simulink model "ACtoAC"  (R2026a)
settings: Solver=ode23t  StopTime=0.05  MaxStep=0.001  RelTol=1e-6  AbsTol=1e-6  EnableMultiTasking=on
libraries: nesl_utility x35, fl_lib x34, ee_lib x17
CloseFcn:
  | try,close(h1_FullWaveBridgeRectifier),end
  | clear h1_FullWaveBridgeRectifier
  | 
  | 
  | clear simlog_FullWaveBridgeRectifier
Description:
  | Full-Wave Bridge Rectifier
settings Model: Creator=The MathWorks, Inc.  LastModifiedBy=MME
settings DebuggingCC: PregeneratedLibrarySubsystemCodeDiagnostic=none
settings HardwareCC: ProdHWDeviceType=32-bit Generic
settings SimscapeCC: SimscapeNominalValues="[{\"value\":\"1\",\"unit\":\"A\"},{\"value\":\"1\",\"unit\":\"bar\"},{\"value\":\"1\",\"unit\":\"cm^2\"},{\"value\":\"1\",\"unit\":\"cm^3/s\"},{\"value\":\"1\",\"unit\":\"kJ/kg\"},{\"value\":\"1\",\"unit\":\"kW\"},{\"value\":\"1\",\"unit\":\"l\"},{\"value\":\"1\",\"unit\":\"N\"},{\"value\":\"1\",\"unit\":\"N*m\"},{\"value\":\"1\",\"unit\":\"V\"}]"  SimscapeLogSimulationStatistics=on  SimscapeLogName=simlog_FullWaveBridgeRectifier

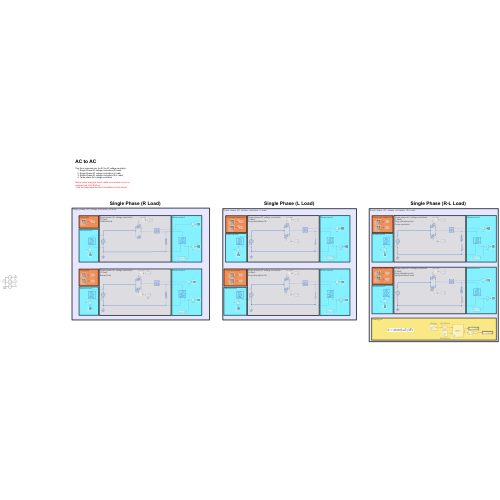
[thumbnail: Simulink's stored preview of the top-level diagram]
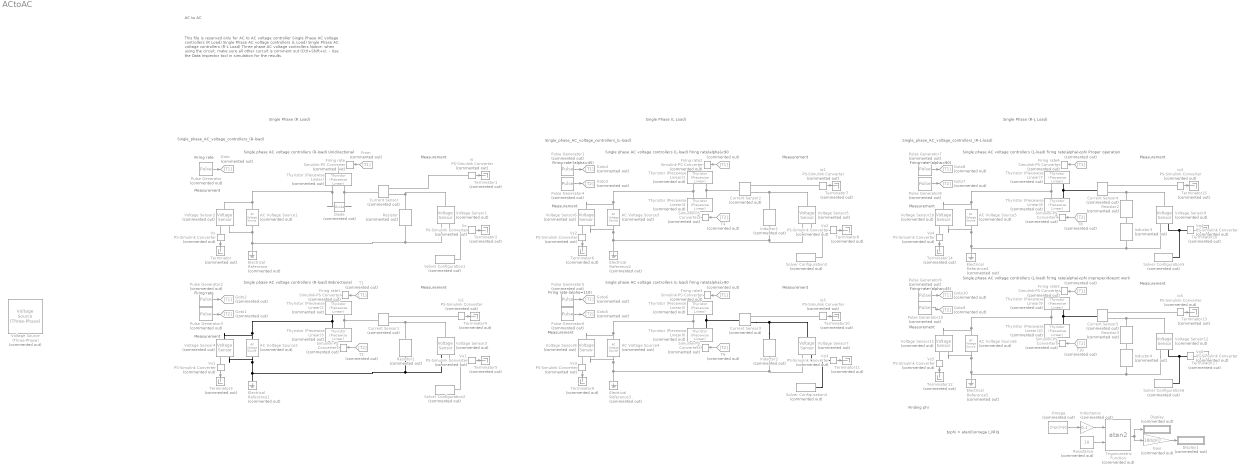
== system ACtoAC ==
  note: $\phi = atan((\omega L)/R)$
  note: Finding phi
  note: Single_phase_AC_voltage_controllers_(L-load)
  note: Single_phase_AC_voltage_controllers_(R-load)
  note: Measurement
  note: Firing rate
  note: Single phase AC voltage controllers
      | (R-load)
      | Unidirectional
  note: This file is reserved only for AC to AC voltage controller
      | Single Phase AC voltage controllers (R Load)
      | Single Phase AC voltage controllers (L Load)
      | Single Phase AC voltage controllers (R-L Load)
      | Three phase AC voltage controllers
      |
      | Notice: when using the circuit, make sure all other curcuit is comment out (Ctrl+Shift+x).
      | - Use the Data Inspector tool in simulation for the results.
  note: AC to AC
  note: Measurement
  note: Measurement
  note: Single phase AC voltage controllers
      | (R-load)
      | Bidirectional
  note: Firing rate
  note: Measurement
  note: Measurement
  note: Single phase AC voltage controllers
      | (L-load)
      | firing rate(alpha)<90
  note: Firing rate (alpha=45)
  note: Measurement
  note: Firing rate (alpha=110)
  note: Measurement
  note: Measurement
  note: Single phase AC voltage controllers
      | (L-load)
      | firing rate(alpha)>90
  note: Single Phase (R Load)
  note: Single Phase (L Load)
  note: Single Phase (R-L Load)
  note: Single_phase_AC_voltage_controllers_(R-L-load)
  note: Firing rate (alpha=90)
  note: Measurement
  note: Measurement
  note: Single phase AC voltage controllers
      | (L-load)
      | firing rate(alpha)<phi
      | Proper operation
  note: Single phase AC voltage controllers
      | (L-load)
      | firing rate(alpha)<phi
      | improper/doesnt work
  note: Measurement
  note: Firing rate (alpha=45)
  note: Measurement
  AC Voltage Source{1..6} (6 alike) : fl_lib/Electrical/Electrical Sources/AC Voltage Source  Commented=on  amp=120*sqrt(2) V  shift=0 deg  frequency=50 Hz
  Current Sensor{,1..5} (6 alike) : fl_lib/Electrical/Electrical Sensors/Current Sensor  Commented=on
  Diode : ee_lib/Semiconductors & Converters/Diode  Commented=on  ModelType=ee.enum.diode.modelType.pwl  TableType=ee.enum.diode.tableType.IfMat  IfMat=[.07, .12, .19, 1.75, 4.24, 7.32, 11.2; .16, .3, .72, 2.14, 5.02, 8.35, 13.12] A  VfMat=[.9, 1.15, 1.25, 1.5, 1.75, 2.17, 2.6, 2.85; .58, .68, .75, 1.1, 1.38, 1.77, 2.27, 2.7] V  TjVec=[25, 125] degC  VfVec=[.5, .7, .9, 1.3, 1.7, 2.1, 2.5] V  IfVec=[.1, .2, .5, 1, 2, 4, 7, 10] A  IrMat=[1e-06, 2e-06, 5e-06, 1e-05, 2.5e-05, 5e-05, .0001; 2e-06, 5e-06, 1e-05, 4e-05, 8e-05, .0002, .0005] A  VrMat=[10, 100, 200, 250, 300, 325, 350; 10, 70, 160, 220, 270, 300, 320] V  VrVec=[10, 20, 40, 50, 70, 80, 100] V  IrVec=[1e-06, 2e-06, 5e-06, 1e-05, 2e-05, 5e-05, .0001] A  Vf=0.6 V  Ron=0.3 Ohm  Goff=1e-8 S  prmExp=ee.enum.diode.expParam.useTwo  I12=[.0137, .545] A  V12=[.6, .7] V  RS=0 Ohm  Tmeas=298.15 K  IS=1e-12 A  ec=1  I1=0.0137 A  V1=0.6 V  N_series=1  N_parallel=1  ZenerEnable=false  Rz=0.3 Ohm  BV=30 V  C_param=ee.enum.diode.capParam.fixed  CJ=0 pF  CJ0=5 pF  Vvec=[.1, 10, 100] V  Cvec=[3.5, 1, .4] pF  VJ=1 V  Mgrad=0.5  FC=0.5  Q_param=ee.enum.diode.recoveryParam.off  iRM=-7.15 A  iF=4 A  didt=-750 A/us  trr_factor=3  trr=115 ns  Qrr=150 nA*s  Vr=-600 V  Ls=150 nH  Erec=0.03 J  TT=50 ns  tau=100 ns  T_param=ee.enum.diode.temperatureParam.off  Tdevice=298.15 K  I1_T2=0.245 A  V1_T2=0.5 V  IS_T2=1.25e-7 A  Tmeas2=125 degC  XTI_param=ee.enum.diode.xtiParam.pn  XTI=3  EG_param=ee.enum.diode.egapParam.material_si  EG=1.11 eV  dBVdT=0 V/K  enable_fault_input=simscape.enum.onoff.off  i_specify=off  i_priority=None  i=0 A  i_nominal_specify=off  i_nominal_value=1  i_nominal_unit=A  v_specify=off  v_priority=None  v=0 V  v_nominal_specify=off  v_nominal_value=1  v_nominal_unit=V  v_capacitor_specify=off  v_capacitor_priority=None  v_capacitor=0 V  v_capacitor_nominal_specify=off  v_capacitor_nominal_value=1  v_capacitor_nominal_unit=V  Qj_specify=off  Qj_priority=High  Qj=0 C  Qj_nominal_specify=off  Qj_nominal_value=1  Qj_nominal_unit=C  i_diode_specify=off  i_diode_priority=None  i_diode=0 A  i_diode_nominal_specify=off  i_diode_nominal_value=1  i_diode_nominal_unit=A  v_diode_specify=off  v_diode_priority=None  v_diode=0 V  v_diode_nominal_specify=off  v_diode_nominal_value=1  v_diode_nominal_unit=V  i_capacitor_specify=off  i_capacitor_priority=None  i_capacitor=0 A  i_capacitor_nominal_specify=off  i_capacitor_nominal_value=1  i_capacitor_nominal_unit=A  fidelity_level=ee.enum.diode.fidelity.includeChargeDyn  rec_loss_model=ee.enum.diode.reverseRecoveryModelTabulateUpTo3D.fixed  ErecVal=0 J  scaleWithIandV=true  ErecMat=zeros(2, 3) J  ErecMat3D=zeros(2, 3, 2) J  TjrecVec=[298.15, 398.15] K  IfrecVec=[.1, 1, 10] A  IrecVal=10 A  VrecVal=10 V  VrecVec=[0, 100] V  tFilter=1 / 1000 / 100 s  thermal_network_parameterization=ee.enum.thermalNetworkTopology.junctionCase  Rth=[0, 10] K/W  Rth_Cauer=[1, 3, 10] K/W  Rth_Foster=[.08, .14, .22, .16] K/W  thermal_mass_parameterization=ee.enum.thermalNetwork.timeconstant  thermal_mass=[0, 1] J/K  thermal_mass_Cauer=[.1, .3, 1] J/K  thermal_mass_Foster=[.001, .005, .05, .5] J/K  thermal_time_constant=[0, 10] s  thermal_time_constant_Cauer=[1, 3, 10] s  thermal_time_constant_Foster=[7e-05, .0007, .01, .08] s  thermal_mass_initial_temperatures=[25, 25] degC  thermal_mass_initial_temperatures_Cauer=[25, 25, 25] degC  junction_thermal_mass=0.01 J/K  Tvec_initial_Foster=[25, 25, 25, 25] degC  no_thermal_network=0  junction_temperature_specify=off  junction_temperature_priority=None  junction_temperature=25 degC  junction_temperature_nominal_specify=off  junction_temperature_nominal_value=1  junction_temperature_nominal_unit=degC
  Display : Display  Commented=on
  Display1 : Display  Commented=on
  Electrical Reference{,1..5} (6 alike) : fl_lib/Electrical/Electrical Elements/Electrical Reference  Commented=on
  Firing rate{,1..5} (6 alike) : nesl_utility/Simulink-PS Converter  Commented=on  PhysicalDomain=network_engine_domain  SubClassName=ps_input  LeftPortType=input  RightPortType=output  PseudoPeriodic=off  Frequencies=[]  NoiseDistribution=none  NoiseParameters=[]  Unit=1  AffineConversion=off  FilteringAndDerivatives=provide  SimscapeFilterOrder=1  InputFilterTimeConstant=0.001  UdotUserProvided=0
  From : From  Commented=on  GotoTag=T1
  Gain : Gain  Commented=on  Gain=180/pi()
  Goto{,2,4,6,8,10} (6 alike) : Goto  Commented=on  GotoTag=T1
  Goto{1,3,5,7,9} (5 alike) : Goto  Commented=on  GotoTag=T2
  Inductance : Gain  Commented=on  Gain=0.1
  Inductor{1..4} (4 alike) : ee_lib/Passive/Inductor  Commented=on  l=1e-1 H  enable_L_tol=ee.enum.toleranceApplication.none  L_tol=20  tol_distribution=ee.enum.toleranceDistribution.uniform  nSigma=4  r=0 Ohm  g=1e-9 1/Ohm  enable_operating_limits=ee.enum.enable.no  operating_limit_action=ee.enum.passive.reportOpLim.warn  max_working_current=1 A  power_rating=1 W  i_L_specify=off  i_L_priority=High  i_L=0 A  i_L_nominal_specify=off  i_L_nominal_value=1  i_L_nominal_unit=A
  Omega : Constant  Commented=on  Value=2*pi()*50
  Pulse Generator : DiscretePulseGenerator  Commented=on  PulseType=Time based  Amplitude=10  Period=0.02  PulseWidth=30  PhaseDelay=0.02*45/360
  Pulse Generator1 : DiscretePulseGenerator  Commented=on  PulseType=Time based  Amplitude=10  Period=0.02  PulseWidth=10  PhaseDelay=0.02*45/360
  Pulse Generator10 : DiscretePulseGenerator  Commented=on  PulseType=Time based  Amplitude=10  Period=0.02  PulseWidth=10  PhaseDelay=0.02*(70+180)/360
  Pulse Generator2 : DiscretePulseGenerator  Commented=on  PulseType=Time based  Amplitude=10  Period=0.02  PulseWidth=30  PhaseDelay=0.02*45/360
  Pulse Generator3 : DiscretePulseGenerator  Commented=on  PulseType=Time based  Amplitude=10  Period=0.02  PulseWidth=30  PhaseDelay=0.02*(45+180)/360
  Pulse Generator4 : DiscretePulseGenerator  Commented=on  PulseType=Time based  Amplitude=10  Period=0.02  PulseWidth=10  PhaseDelay=0.02*(45+180)/360
  Pulse Generator5 : DiscretePulseGenerator  Commented=on  PulseType=Time based  Amplitude=10  Period=0.02  PulseWidth=10  PhaseDelay=0.02*110/360
  Pulse Generator6 : DiscretePulseGenerator  Commented=on  PulseType=Time based  Amplitude=10  Period=0.02  PulseWidth=10  PhaseDelay=0.02*(110+180)/360
  Pulse Generator7 : DiscretePulseGenerator  Commented=on  PulseType=Time based  Amplitude=10  Period=0.02  PulseWidth=10  PhaseDelay=0.02*90/360
  Pulse Generator8 : DiscretePulseGenerator  Commented=on  PulseType=Time based  Amplitude=10  Period=0.02  PulseWidth=10  PhaseDelay=0.02*(90+180)/360
  Pulse Generator9 : DiscretePulseGenerator  Commented=on  PulseType=Time based  Amplitude=10  Period=0.02  PulseWidth=10  PhaseDelay=0.02*70/360
  Resistance : Constant  Commented=on  Value=10
  Resistor : fl_lib/Electrical/Electrical Elements/Resistor  Commented=on  R=1 Ohm  i_specify=off  i_priority=None  i=0 A  i_nominal_specify=off  i_nominal_value=1  i_nominal_unit=A  v_specify=off  v_priority=None  v=0 V  v_nominal_specify=off  v_nominal_value=1  v_nominal_unit=V
  Resistor1 : fl_lib/Electrical/Electrical Elements/Resistor  Commented=on  R=1 Ohm  i_specify=off  i_priority=None  i=0 A  i_nominal_specify=off  i_nominal_value=1  i_nominal_unit=A  v_specify=off  v_priority=None  v=0 V  v_nominal_specify=off  v_nominal_value=1  v_nominal_unit=V
  Resistor2 : fl_lib/Electrical/Electrical Elements/Resistor  Commented=on  R=10 Ohm  i_specify=off  i_priority=None  i=0 A  i_nominal_specify=off  i_nominal_value=1  i_nominal_unit=A  v_specify=off  v_priority=None  v=0 V  v_nominal_specify=off  v_nominal_value=1  v_nominal_unit=V
  Resistor3 : fl_lib/Electrical/Electrical Elements/Resistor  Commented=on  R=10 Ohm  i_specify=off  i_priority=None  i=0 A  i_nominal_specify=off  i_nominal_value=1  i_nominal_unit=A  v_specify=off  v_priority=None  v=0 V  v_nominal_specify=off  v_nominal_value=1  v_nominal_unit=V
  Simulink-PS Converter{1..5} (5 alike) : nesl_utility/Simulink-PS Converter  Commented=on  PhysicalDomain=network_engine_domain  SubClassName=ps_input  LeftPortType=input  RightPortType=output  PseudoPeriodic=off  Frequencies=[]  NoiseDistribution=none  NoiseParameters=[]  Unit=1  AffineConversion=off  FilteringAndDerivatives=provide  SimscapeFilterOrder=1  InputFilterTimeConstant=0.001  UdotUserProvided=0
  Solver Configuration{1..6} (6 alike) : nesl_utility/Solver Configuration  Commented=on  PhysicalDomain=network_engine_domain  SubClassName=solver  LeftPortType=input  RightPortType=generic  Tones=[]  Harmonics=[]  SimulateNoise=off  Profile=off  UseLocalSampling=off  EnableSwitchedLinearOptims=on  FrequencyDomain=off  UseCCode=off  RelTol=0.001  AbsTol=1e-06  MinStep=1e-09  ToWorkspace=off  RevertToSquareIcSolve=off  NumHomotopyIterations=100  PhasorMode=off  PhasorModeNumHarmonics=1  ConsistencySolver=NEWTON_XTOL_AFTER_FTOL  CanonicalOrdering=UNORDERED  OptimizeIntermediates=UNOPTIMIZED  IndexReductionMethod=DerivativeReplacement  DoDC=off  ResidualTolerance=1e-9  ConsistencyTolSource=GLOBAL  ConsistencyAbsTol=0.001  ConsistencyRelTol=0.001  ConsistencyTolFactor=0.001  UseLocalSolver=off  LocalSolverChoice=NE_BACKWARD_EULER_ADVANCER  ResolveIndetEquations=on  FunctionEvalNumThread=1  LocalSolverSampleTime=.001  DoFixedCost=off  MaxNonlinIter=3  MaxModeIter=2  ComputeImpulses=off  ImpulseIterations=2  LinearAlgebra=auto  LinearAlgebraNumThread=0  EquationFormulation=NE_TIME_EF  DelaysMemoryBudget=1024  AutomaticFiltering=on  FilteringTimeConstant=0.001  PartitionStorageMethod=AS_NEEDED  PartitionMemoryBudget=1024  PartitionMethod=FAST  MultibodyUseLocalSolver=off  MultibodyLocalSolverChoice=ODE1  MultibodyLocalSolverSampleTime=0.001
  T{1,3,5,7,9} (5 alike) : From  Commented=on  GotoTag=T1
  T{2,4,6,8,10} (5 alike) : From  Commented=on  GotoTag=T2
  Terminator{,1..17} (18 alike) : Terminator  Commented=on
  Thyristor (Piecewise Linear){,1..10} (11 alike) : ee_lib/Semiconductors & Converters/Thyristor (Piecewise Linear)  Commented=on  port_option=ee.enum.controlport.ps  Vf=0.8 V  Ron=0.001 Ohm  Goff=1e-5 1/Ohm  Vgt=6 V  Ih=1 A  diode_param=ee.enum.semiconductors.protectionDiode.external  diode_Vf=0.8 V  diode_Ron=0.001 Ohm  diode_Goff=1e-5 1/Ohm  diode_C=50e-9 F  diode_iRM=-235 A  diode_iF=300 A  diode_idot=-50 A/us  diode_trr_param=ee.enum.converters.diodetrr.trr_factor  diode_trr_factor=3  diode_trr=15 us  diode_Qrr=1500 s*uA  iak_specify=off  iak_priority=None  iak=0 A  iak_nominal_specify=off  iak_nominal_value=1  iak_nominal_unit=A  vak_specify=off  vak_priority=None  vak=0 V  vak_nominal_specify=off  vak_nominal_value=1  vak_nominal_unit=V  vgk_specify=off  vgk_priority=None  vgk=0 V  vgk_nominal_specify=off  vgk_nominal_value=1  vgk_nominal_unit=V  thermal_loss_option=ee.enum.converters.thermalLossOption.constantvalues  Von_data=[0, .1, .6, .8, 1, 1.3, 1.6, 2, 2.4; 0, .1, .7, 1, 1.2, 1.5, 1.9, 2.4, 2.8] V  Tj=[298.15, 398.15] K  Iout_data=[0, .1, 1, 5, 10, 20, 40, 70, 100] A  Eon_data=[0, .0024, .024, .12, .2, .48, 1.04, 2.16, 3.24; 0, .003, .03, .15, .25, .6, 1.3, 2.7, 4.05] * 1e-3 J  Tj_loss=[298.15, 398.15] K  Iout_data_loss=[0, .1, 1, 5, 10, 20, 40, 70, 100] A  Eon_scalar=22.86e-3 J  Eoff_natural_commutation=10e-3 J  Voff=300 V  Iout_scalar=600 A  onCurrentMeasDelay=1e-4 s  diodeModelType=ee.enum.converters.diodeModelType.pwl  diodeTableType=ee.enum.diode.tableType.IfMat  diode_IfMat=[.07, .12, .19, 1.75, 4.24, 7.32, 11.2; .16, .3, .72, 2.14, 4.02, 6.35, 9.12] A  diode_VfMat=[.9, 1.15, 1.25, 1.5, 1.75, 2.17, 2.6, 2.85; .58, .68, .75, 1.1, 1.38, 1.77, 2.27, 2.7] V  diode_TjVec=[25, 125] degC  diode_VfVec=[.5, .7, .9, 1.3, 1.7, 2.1, 2.5] V  diode_IfVec=[.1, .2, .5, 1, 2, 4, 7, 10] A  diode_rec_loss_model=ee.enum.diode.reverseRecoveryModel.fixed  diode_ErecVal=0 J  diode_scaleWithIandV=true  diode_ErecMat=zeros(2, 3) J  diode_TjrecVec=[298.15, 398.15] K  diode_IfrecVec=[.1, 1, 10] A  diode_IrecVal=10 A  diode_VrecVal=10 V  diode_tFilter=1 / 1000 / 100 s  thermal_network_parameterization=ee.enum.thermalNetworkTopology.external  Rth=[.08, .5] K/W  Rth_Cauer=[.08, .1, .5] K/W  Rth_Foster=[.08, .14, .22, .16] K/W  thermal_mass_parameterization=ee.enum.thermalNetwork.timeconstant  thermal_mass=[.01, .5] J/K  thermal_mass_Cauer=[.01, .1, .5] J/K  thermal_mass_Foster=[.001, .005, .05, .5] J/K  thermal_time_constant=[.001, .2] s  thermal_time_constant_Cauer=[.001, .1, .2] s  thermal_time_constant_Foster=[7e-05, .0007, .01, .08] s  thermal_mass_initial_temperatures=[25, 25] degC  thermal_mass_initial_temperatures_Cauer=[25, 25, 25] degC  junction_thermal_mass=0.01 J/K  Tvec_initial_Foster=[25, 25, 25, 25] degC  junction_temperature_specify=off  junction_temperature_priority=None  junction_temperature=25 degC  junction_temperature_nominal_specify=off  junction_temperature_nominal_value=1  junction_temperature_nominal_unit=degC  Qj_specify=off  Qj_priority=None  Qj=0 W  Qj_nominal_specify=off  Qj_nominal_value=1  Qj_nominal_unit=W  accumulatedSwitchingLosses_specify=off  accumulatedSwitchingLosses_priority=None  accumulatedSwitchingLosses=0 J
  Trigonometric Function : Trigonometry  Commented=on  Operator=atan2
  Vo{,1..5} (6 alike) : nesl_utility/PS-Simulink Converter  Commented=on  PhysicalDomain=network_engine_domain  SubClassName=ps_output  LeftPortType=input  RightPortType=output  PseudoPeriodic=off  Frequencies=[]  VectorFormat=inherit  Unit=inherit  AffineConversion=off
  Voltage Source (Three-Phase) : ee_lib/Sources/Voltage Source (Three-Phase)  Commented=on  vline_rms=sqrt(3) * 325 / sqrt(2) V  shift=0 deg  freq=50 Hz  impedance_option=1  SShortCircuit=1e6 A*V  XR=15  R=0.01 Ohm  L=3.97e-4 H  harmonic_option=0  harmonic_orders=[5, 7, 11, 13]  harmonic_ratios=[.1, .1, .1, .1]  G_parasitic=0 1/Ohm  I_specify=off  I_priority=None  I=[0, 0, 0] A  I_nominal_specify=off  I_nominal_value=1  I_nominal_unit=A
  Voltage Sensor{1..12} (12 alike) : fl_lib/Electrical/Electrical Sensors/Voltage Sensor  Commented=on
  Vs{,1..5} (6 alike) : nesl_utility/PS-Simulink Converter  Commented=on  PhysicalDomain=network_engine_domain  SubClassName=ps_output  LeftPortType=input  RightPortType=output  PseudoPeriodic=off  Frequencies=[]  VectorFormat=inherit  Unit=inherit  AffineConversion=off
  io{,1..5} (6 alike) : nesl_utility/PS-Simulink Converter  Commented=on  PhysicalDomain=network_engine_domain  SubClassName=ps_output  LeftPortType=input  RightPortType=output  PseudoPeriodic=off  Frequencies=[]  VectorFormat=inherit  Unit=inherit  AffineConversion=off
  wires:
  From/1 -> Firing rate/1
  Pulse Generator/1 -> Goto/1
  Vo/1 -> Terminator2/1
  io/1 -> Terminator1/1
  Vs/1 -> Terminator/1
  io1/1 -> Terminator4/1
  Vs1/1 -> Terminator3/1
  Pulse Generator3/1 -> Goto1/1
  T1/1 -> Firing rate1/1
  Vo1/1 -> Terminator5/1
  T2/1 -> Simulink-PS Converter1/1
  Pulse Generator2/1 -> Goto2/1
  Vo2/1 -> Terminator8/1
  T3/1 -> Firing rate2/1
  T4/1 -> Simulink-PS Converter2/1
  io2/1 -> Terminator7/1
  Vs2/1 -> Terminator6/1
  Pulse Generator4/1 -> Goto3/1
  Pulse Generator1/1 -> Goto4/1
  Vo3/1 -> Terminator11/1
  Pulse Generator6/1 -> Goto5/1
  Vs3/1 -> Terminator9/1
  T6/1 -> Simulink-PS Converter3/1
  io3/1 -> Terminator10/1
  Pulse Generator5/1 -> Goto6/1
  T5/1 -> Firing rate3/1
  Vo4/1 -> Terminator16/1
  Pulse Generator8/1 -> Goto7/1
  Vs4/1 -> Terminator14/1
  T8/1 -> Simulink-PS Converter4/1
  io4/1 -> Terminator15/1
  Pulse Generator7/1 -> Goto8/1
  T7/1 -> Firing rate4/1
  Trigonometric Function/1 -> Display/1, Gain/1
  Omega/1 -> Inductance/1
  Inductance/1 -> Trigonometric Function/1
  Resistance/1 -> Trigonometric Function/2
  Gain/1 -> Display1/1
  io5/1 -> Terminator13/1
  Vs5/1 -> Terminator12/1
  T10/1 -> Simulink-PS Converter5/1
  Pulse Generator9/1 -> Goto10/1
  Pulse Generator10/1 -> Goto9/1
  Vo5/1 -> Terminator17/1
  T9/1 -> Firing rate5/1
  connections:
  AC Voltage Source1/RConn1 -- Voltage Sensor2/RConn2 -- Electrical Reference/LConn1 -- Voltage Sensor1/RConn2 -- Resistor/RConn1
  AC Voltage Source1/LConn1 -- Diode/RConn1 -- Thyristor (Piecewise Linear)/RConn1 -- Voltage Sensor2/LConn1
  Current Sensor/LConn1 -- Diode/LConn1 -- Thyristor (Piecewise Linear)/RConn2
  Solver Configuration1/RConn1 -- Vo/LConn1 -- Voltage Sensor1/RConn1
  io/LConn1 -- Current Sensor/RConn1
  Vs/LConn1 -- Voltage Sensor2/RConn1
  Resistor1/RConn1 -- Electrical Reference1/LConn1 -- Voltage Sensor4/RConn2 -- AC Voltage Source2/RConn1 -- Voltage Sensor3/RConn2
  Voltage Sensor4/LConn1 -- AC Voltage Source2/LConn1 -- Thyristor (Piecewise Linear)3/RConn2 -- Thyristor (Piecewise Linear)2/RConn1
  Current Sensor1/LConn1 -- Thyristor (Piecewise Linear)3/RConn1 -- Thyristor (Piecewise Linear)2/RConn2
  Solver Configuration2/RConn1 -- Vo1/LConn1 -- Voltage Sensor3/RConn1
  Firing rate1/RConn1 -- Thyristor (Piecewise Linear)2/LConn1
  Vs1/LConn1 -- Voltage Sensor4/RConn1
  io1/LConn1 -- Current Sensor1/RConn1
  Simulink-PS Converter1/RConn1 -- Thyristor (Piecewise Linear)3/LConn1
  Firing rate/RConn1 -- Thyristor (Piecewise Linear)/LConn1
  Resistor/LConn1 -- Current Sensor/RConn2 -- Voltage Sensor1/LConn1
  Resistor1/LConn1 -- Current Sensor1/RConn2 -- Voltage Sensor3/LConn1
  Thyristor (Piecewise Linear)4/RConn2 -- Thyristor (Piecewise Linear)1/RConn1 -- Voltage Sensor6/LConn1 -- AC Voltage Source3/LConn1
  Solver Configuration3/RConn1 -- Vo2/LConn1 -- Voltage Sensor5/RConn1
  Current Sensor2/LConn1 -- Thyristor (Piecewise Linear)4/RConn1 -- Thyristor (Piecewise Linear)1/RConn2
  Voltage Sensor5/RConn2 -- Electrical Reference2/LConn1 -- Voltage Sensor6/RConn2 -- AC Voltage Source3/RConn1 -- Inductor1/RConn1
  Current Sensor2/RConn2 -- Voltage Sensor5/LConn1 -- Inductor1/LConn1
  Simulink-PS Converter2/RConn1 -- Thyristor (Piecewise Linear)4/LConn1
  Vs2/LConn1 -- Voltage Sensor6/RConn1
  Firing rate2/RConn1 -- Thyristor (Piecewise Linear)1/LConn1
  io2/LConn1 -- Current Sensor2/RConn1
  Inductor2/LConn1 -- Current Sensor3/RConn2 -- Voltage Sensor7/LConn1
  AC Voltage Source4/RConn1 -- Voltage Sensor7/RConn2 -- Inductor2/RConn1 -- Electrical Reference3/LConn1 -- Voltage Sensor8/RConn2
  Voltage Sensor7/RConn1 -- Solver Configuration4/RConn1 -- Vo3/LConn1
  AC Voltage Source4/LConn1 -- Thyristor (Piecewise Linear)6/RConn2 -- Thyristor (Piecewise Linear)5/RConn1 -- Voltage Sensor8/LConn1
  Thyristor (Piecewise Linear)5/RConn2 -- Current Sensor3/LConn1 -- Thyristor (Piecewise Linear)6/RConn1
  Vs3/LConn1 -- Voltage Sensor8/RConn1
  io3/LConn1 -- Current Sensor3/RConn1
  Firing rate3/RConn1 -- Thyristor (Piecewise Linear)5/LConn1
  Simulink-PS Converter3/RConn1 -- Thyristor (Piecewise Linear)6/LConn1
  Voltage Sensor9/RConn1 -- Solver Configuration5/RConn1 -- Vo4/LConn1
  Current Sensor4/RConn2 -- Resistor2/LConn1 -- Voltage Sensor9/LConn1
  AC Voltage Source5/RConn1 -- Electrical Reference4/LConn1 -- Inductor3/RConn1 -- Voltage Sensor9/RConn2 -- Voltage Sensor10/RConn2
  AC Voltage Source5/LConn1 -- Thyristor (Piecewise Linear)8/RConn2 -- Thyristor (Piecewise Linear)7/RConn1 -- Voltage Sensor10/LConn1
  Thyristor (Piecewise Linear)7/RConn2 -- Current Sensor4/LConn1 -- Thyristor (Piecewise Linear)8/RConn1
  Vs4/LConn1 -- Voltage Sensor10/RConn1
  Simulink-PS Converter4/RConn1 -- Thyristor (Piecewise Linear)8/LConn1
  io4/LConn1 -- Current Sensor4/RConn1
  Firing rate4/RConn1 -- Thyristor (Piecewise Linear)7/LConn1
  Inductor3/LConn1 -- Resistor2/RConn1
  AC Voltage Source6/LConn1 -- Voltage Sensor11/LConn1 -- Thyristor (Piecewise Linear)10/RConn2 -- Thyristor (Piecewise Linear)9/RConn1
  Thyristor (Piecewise Linear)9/RConn2 -- Current Sensor5/LConn1 -- Thyristor (Piecewise Linear)10/RConn1
  AC Voltage Source6/RConn1 -- Electrical Reference5/LConn1 -- Inductor4/RConn1 -- Voltage Sensor12/RConn2 -- Voltage Sensor11/RConn2
  Current Sensor5/RConn2 -- Resistor3/LConn1 -- Voltage Sensor12/LConn1
  Voltage Sensor12/RConn1 -- Solver Configuration6/RConn1 -- Vo5/LConn1
  Simulink-PS Converter5/RConn1 -- Thyristor (Piecewise Linear)10/LConn1
  Firing rate5/RConn1 -- Thyristor (Piecewise Linear)9/LConn1
  io5/LConn1 -- Current Sensor5/RConn1
  Inductor4/LConn1 -- Resistor3/RConn1
  Vs5/LConn1 -- Voltage Sensor11/RConn1
